simulink model "emldemo_process_signal"  (Simulink 7.6)
settings: Solver=FixedStepDiscrete  StartTime=0.0  StopTime=1  RelTol=1e-3
libraries: simulink x1
settings Model: Creator=The MathWorks Inc.
settings DebuggingCC: StrictBusMsg=Warning
settings SFSimCC: SimParseCustomCode=off

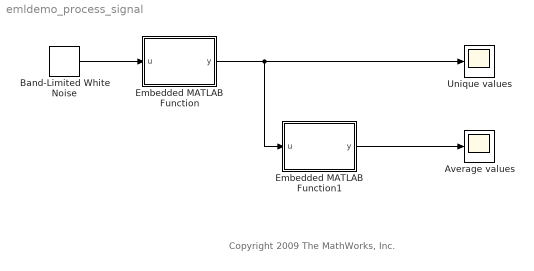
== system emldemo_process_signal ==
  note: Copyright 2009 The MathWorks, Inc.
  Average values : Scope
  Band-Limited White Noise : simulink/Sources/Band-Limited White Noise  SystemSampleTime=-1  Cov=[0.1 0.2 0.3 0.4 0.5 0.6 0.1 0.2 0.3]  Ts=0.1  seed=[2223334]
  Embedded MATLAB Function : Stateflow chart  TreatAsAtomicUnit=on
  Embedded MATLAB Function1 : Stateflow chart  TreatAsAtomicUnit=on
  Unique values : Scope
  wires:
  Band-Limited White Noise/1 -> Embedded MATLAB Function/1(u)
  Embedded MATLAB Function/1(y) -> Unique values/1, Embedded MATLAB Function1/1(u)
  Embedded MATLAB Function1/1(y) -> Average values/1

== matlab function Embedded MATLAB Function1 ==
  data: u input double; y output double size=[1 9]
function y = avg(u)
%#eml

if numel(u) == 1
    y = u;
else
    k = numel(u)/2;
    if k ~= floor(k)
        u = u(2:numel(u));
    end
    y = emldemo_navg(u,2);
end

== matlab function Embedded MATLAB Function ==
  data: u input double; y output double size=[1 9]
function y = uniquify(u)
%#eml

y = emldemo_uniquetol(u,0.2);
